simulink model "fivebar"  (R2018a)
settings: Solver=FixedStepAuto  StartTime=0.0  StopTime=1  FixedStep=10^-3  RelTol=1e-3  EnableMultiTasking=on
values from neighbouring files (symbols this model uses):
  ADAMS_cwd = '\\data-pfe\xshi2017\.Bureau\LAB3'    [Controls_Plant_6.m]    (also in Controls_Plant_7.m; Controls_Plant_8.m)
  ADAMS_exec = ''    [Controls_Plant_6.m]    (also in Controls_Plant_7.m; Controls_Plant_8.m)
  ADAMS_host = 'pc-b101-15.eleves.ecn'    [Controls_Plant_6.m]    (also in Controls_Plant_7.m; Controls_Plant_8.m)
  ADAMS_init = ''    [Controls_Plant_6.m]    (also in Controls_Plant_7.m; Controls_Plant_8.m)
  ADAMS_inputs = 'q11!q21'    [Controls_Plant_6.m]    (also in Controls_Plant_7.m; Controls_Plant_8.m)
  ADAMS_outputs = 'A13x!A13y!A13xd!A13yd!A13xdd!A13ydd!q12!q22!q13!q12d!q22d!q13d!q12dd!q22dd!q13dd!tau1!tau2'    [Controls_Plant_6.m]    (also in Controls_Plant_7.m; Controls_Plant_8.m)
  ADAMS_prefix = 'Controls_Plant_6'    [Controls_Plant_6.m]    (also in Controls_Plant_7.m = 'Controls_Plant_7'; Controls_Plant_8.m = 'Controls_Plant_8')
  ADAMS_static = 'no'    [Controls_Plant_6.m]    (also in Controls_Plant_7.m; Controls_Plant_8.m)
  ADAMS_sysdir = 'D:\Appli\Adams\'    [Controls_Plant_6.m]    (also in Controls_Plant_7.m; Controls_Plant_8.m)
settings Model: Creator=dsix  LastModifiedBy=xshi2017
settings DataIOCC: LimitDataPoints=on  SaveFormat=Array
settings OptimizationCC: LifeSpan=inf
settings DebuggingCC: SFUnexpectedBacktrackingDiag=warning  SFNoUnconditionalDefaultTransitionDiag=warning  SFExecutionAtInitializationDiag=none
settings HardwareCC: ProdBitPerPointer=32  ProdBitPerSizeT=32  ProdBitPerPtrDiffT=32  ProdLargestAtomicFloat=None  ProdIntDivRoundTo=Undefined  ProdEndianess=Unspecified  ProdWordSize=32  ProdHWDeviceType=32-bit Generic
settings ModelReferenceCC: PropagateSignalLabelsOutOfModel=off
settings CodeAppCC: StateflowObjectComments=on
settings GRTTargetCC: TargetLangStandard=C89/C90 (ANSI)  GeneratePreprocessorConditionals=Disable all
settings ConfigComp: CovMetricSettings=dw  CovHtmlReporting=on  CovSaveCumulativeToWorkspaceVar=on  CovSaveSingleToWorkspaceVar=on  CovExternalEMLEnable=off

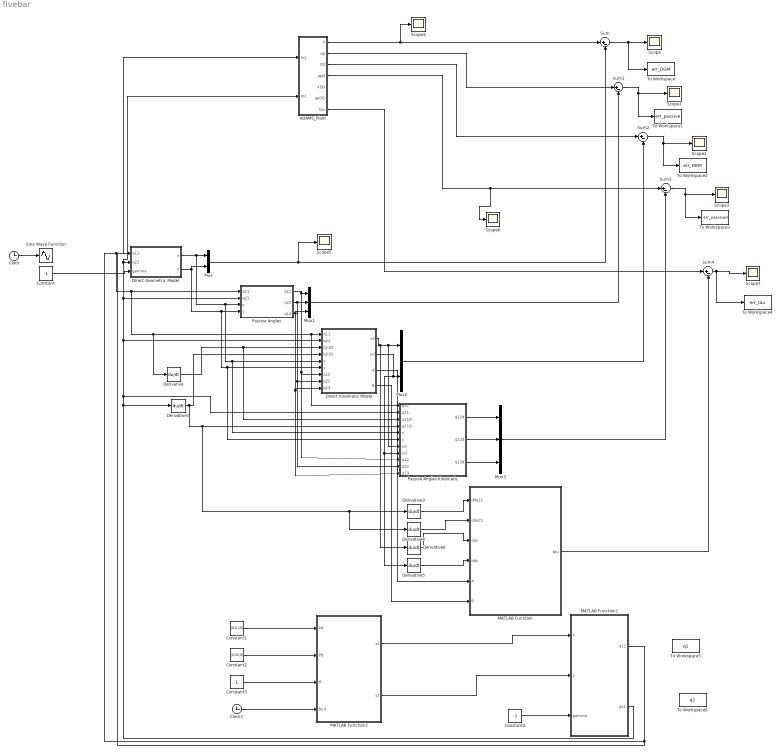
== system fivebar ==
  ADAMS_Plant : Subsystem
  Clock : Clock
  Clock1 : Clock
  Constant : Constant  Value=-1
  Constant1 : Constant  Value=[0;0.15]
  Constant2 : Constant  Value=[0.05;0]
  Constant3 : Constant
  Constant4 : Constant  Value=-1
  Derivative{,1,3..6} (6 alike) : Derivative
  Direct Geometric Model : MATLAB Function  TreatAsAtomicUnit=on
  Direct Kinematic Model : MATLAB Function  TreatAsAtomicUnit=on
  MATLAB Function : MATLAB Function  TreatAsAtomicUnit=on
  MATLAB Function1 : MATLAB Function  TreatAsAtomicUnit=on
  MATLAB Function2 : MATLAB Function  TreatAsAtomicUnit=on
  Mux : Mux  Inputs=2
  Mux1 : Mux  Inputs=3
  Mux2 : Mux  Inputs=2
  Mux3 : Mux  Inputs=3
  Passive Angles : MATLAB Function  TreatAsAtomicUnit=on
  Passive Angles Kinematic : MATLAB Function  TreatAsAtomicUnit=on
  Scope{,1..7} (8 alike) : Scope
  Sine Wave Function : Sin  TimeSource=Use external signal  SampleTime=0
  Sum{,1..4} (5 alike) : Sum  Inputs=|+-
  To Workspace : ToWorkspace  VariableName=err_DGM  SaveFormat=Timeseries  SampleTime=-1
  To Workspace1 : ToWorkspace  VariableName=err_passive  SaveFormat=Timeseries  SampleTime=-1
  To Workspace2 : ToWorkspace  VariableName=err_DKM  SaveFormat=Timeseries  SampleTime=-1
  To Workspace3 : ToWorkspace  VariableName=err_passived  SaveFormat=Timeseries  SampleTime=-1
  To Workspace4 : ToWorkspace  VariableName=err_tau  SaveFormat=Timeseries  SampleTime=-1
  To Workspace5 : ToWorkspace  VariableName=q1  SaveFormat=Timeseries  SampleTime=-1
  To Workspace6 : ToWorkspace  VariableName=q2  SaveFormat=Timeseries  SampleTime=-1
  wires:
  ADAMS_Plant/1(X) -> Scope4/1, Sum/1
  Sum/1 -> To Workspace/1, Scope/1
  Direct Geometric Model/1(x) -> Direct Kinematic Model/5(x), Passive Angles Kinematic/5(x), Passive Angles/3(x), Mux/1
  Direct Geometric Model/2(y) -> Mux/2, Passive Angles Kinematic/6(y), Direct Kinematic Model/6(y), Passive Angles/4(y)
  Mux/1 -> Scope5/1, Sum/2
  Passive Angles/1(q12) -> Passive Angles Kinematic/9(q12), Direct Kinematic Model/7(q12), Mux1/1
  Passive Angles/2(q22) -> Passive Angles Kinematic/10(q22), Direct Kinematic Model/8(q22), Mux1/2
  Passive Angles/3(q13) -> Passive Angles Kinematic/11(q13), Direct Kinematic Model/9(q13), Mux1/3
  ADAMS_Plant/2(qp) -> Sum1/1
  Mux1/1 -> Sum1/2
  Sum1/1 -> To Workspace1/1, Scope1/1
  Direct Kinematic Model/1(xd) -> Derivative6/1, Passive Angles Kinematic/7(xd), Mux2/1
  Direct Kinematic Model/2(yd) -> Passive Angles Kinematic/8(yd), Derivative5/1, Mux2/2
  Sum2/1 -> To Workspace2/1, Scope2/1
  Mux2/1 -> Sum2/2
  ADAMS_Plant/3(XD) -> Sum2/1
  Passive Angles Kinematic/1(q12d) -> Mux3/1
  Passive Angles Kinematic/2(q22d) -> Mux3/2
  Passive Angles Kinematic/3(q13d) -> Mux3/3
  Sum3/1 -> To Workspace3/1, Scope3/1
  Mux3/1 -> Sum3/2
  ADAMS_Plant/4(qpD) -> Scope6/1, Sum3/1
  MATLAB Function1/1(q11) -> Direct Geometric Model/1(q11), Derivative/1, Passive Angles Kinematic/1(q11), Direct Kinematic Model/1(q11), Passive Angles/1(q11), ADAMS_Plant/1(In1)
  Derivative/1 -> Passive Angles Kinematic/3(q11D), Direct Kinematic Model/3(q11D)
  Derivative1/1 -> Derivative4/1, Derivative3/1, Passive Angles Kinematic/4(q21D), Direct Kinematic Model/4(q21D)
  Derivative3/1 -> MATLAB Function/1(ddq11)
  Derivative5/1 -> MATLAB Function/4(ddy)
  Derivative6/1 -> MATLAB Function/3(ddx)
  Direct Kinematic Model/4(B) -> MATLAB Function/6(B)
  Direct Kinematic Model/3(A) -> MATLAB Function/5(A)
  ADAMS_Plant/7(tau) -> Sum4/1
  MATLAB Function/1(tau) -> Sum4/2
  Sum4/1 -> To Workspace4/1, Scope7/1
  Derivative4/1 -> MATLAB Function/2(ddq21)
  Constant1/1 -> MATLAB Function2/1(PA)
  Constant2/1 -> MATLAB Function2/2(PB)
  Constant3/1 -> MATLAB Function2/3(tf)
  Clock1/1 -> MATLAB Function2/4(tout)
  Constant4/1 -> MATLAB Function1/3(gamma)
  Clock/1 -> Sine Wave Function/1
  MATLAB Function2/2(yt) -> MATLAB Function1/2(y)
  MATLAB Function2/1(xt) -> MATLAB Function1/1(x)
  Constant/1 -> Direct Geometric Model/3(gamma)
  MATLAB Function1/2(q21) -> Derivative1/1, Passive Angles Kinematic/2(q21), Direct Kinematic Model/2(q21), Passive Angles/2(q21), ADAMS_Plant/2(In2), Direct Geometric Model/2(q21)

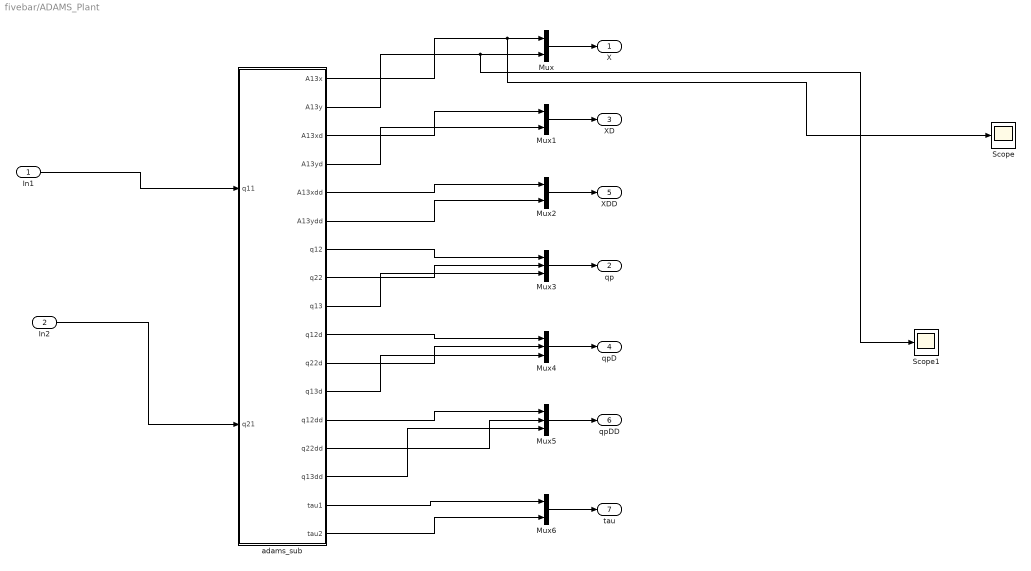
== system fivebar/ADAMS_Plant ==
  In1 : Inport
  In2 : Inport  Port=2
  Mux{,1..2,6} (4 alike) : Mux  Inputs=2
  Mux3 : Mux  Inputs=3
  Mux4 : Mux  Inputs=3
  Mux5 : Mux  Inputs=3
  Scope : Scope
  Scope1 : Scope
  adams_sub : Subsystem
  X : Outport
  qp : Outport  Port=2
  XD : Outport  Port=3
  qpD : Outport  Port=4
  XDD : Outport  Port=5
  qpDD : Outport  Port=6
  tau : Outport  Port=7
  wires:
  Mux1/1 -> XD/1
  Mux/1 -> X/1
  Mux2/1 -> XDD/1
  Mux5/1 -> qpDD/1
  Mux4/1 -> qpD/1
  Mux3/1 -> qp/1
  Mux6/1 -> tau/1
  In1/1 -> adams_sub/1(q11)
  In2/1 -> adams_sub/2(q21)
  adams_sub/1("A13x  ") -> Scope/1, Mux/1
  adams_sub/2("A13y  ") -> Scope1/1, Mux/2
  adams_sub/3("A13xd ") -> Mux1/1
  adams_sub/4("A13yd ") -> Mux1/2
  adams_sub/5(A13xdd) -> Mux2/1
  adams_sub/6(A13ydd) -> Mux2/2
  adams_sub/7("q12   ") -> Mux3/1
  adams_sub/8("q22   ") -> Mux3/2
  adams_sub/9("q13   ") -> Mux3/3
  adams_sub/10("q12d  ") -> Mux4/1
  adams_sub/11("q22d  ") -> Mux4/2
  adams_sub/12("q13d  ") -> Mux4/3
  adams_sub/13("q12dd ") -> Mux5/1
  adams_sub/14("q22dd ") -> Mux5/2
  adams_sub/15("q13dd ") -> Mux5/3
  adams_sub/16("tau1  ") -> Mux6/1
  adams_sub/17("tau2  ") -> Mux6/2

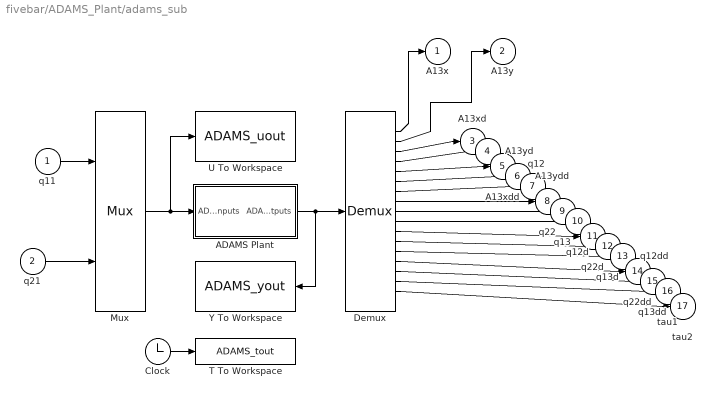
== system fivebar/ADAMS_Plant/adams_sub ==
  q11 : Inport
  q21 : Inport  Port=2
  ADAMS Plant : Subsystem  LoadFcn=|  InitFcn=clear mex  mask(Adams Plant){exevie=ADAMS_sysdir, nam_in=ADAMS_inputs, namout=ADAMS_outputs, nampre=ADAMS_prefix, outfil=ADAMS_prefix, exesol=ADAMS_exec, stat=ADAMS_static, inicmd=[ADAMS_init], exetyp=C++, comtyp=PIPE(DDE), workdir=ADAMS_cwd, ada_host=ADAMS_host, modani=interactive, modsim=discrete, dft=no, simulink_lead_cosim=yes, pin_interp_order=0, pout_extrap_order=0, pin_extrap_order=0, pout_interp_order=0, dt_out=0.005, o_rate=1, more=off}
      | %check based on dialog box setting for when setting by popup menu                                             
      | if exist('ADAMS_solver_type')                                                                                 
      |   if strcmp(ADAMS_solver_type,'C++')                                                                          
      |     set_param(gcb,'exetyp','C++');                                                                            
      |   else                                                                                                        
      |     set_param(gcb,'exetyp','Fortran');                                                                        
      |   end                                                                                                         
      | else                                                                                                          
      |   set_param(gcb,'exetyp','C++');                                                                              
      | end                                                                                                           
      | %set the mode if using acar_solver                                                                            
      | %REQUIRED HERE BECAUSE BELOW CAUSES MDLTERMINATE TO BE CALLED 2 TIMES IN MIDDLE OF SIMULATION WHEN SET IN MASK
      |                                                                                                               
      | %enable the direct feedthrough, sim mode, anim mode parameters by default                                     
      |                                                                                                               
      | if exist('set_some_params_states')                                                                            
      |                                                                                                               
      |   set_some_params_states({'dft','modsim','modani'},{'on','on','on'},'MaskEnables',gcb)                        
      |   %turn on direct feedthrough option                                                                          
      |   set_some_params_states({'dft'},{'on'},'MaskVisibilities',gcb)                                               
      |                                                                                                               
      |  end                                                                                                          
      |                                                                                                               
      |                                                                                                               
      | if exist('ADAMS_exec')                                                                                        
      |   if and(strcmp(get_param(gcb,'exesol'),'ADAMS_exec'),strcmp(ADAMS_exec,'acar_solver'))                       
      |     %set the sim mode to discrete -- only supported mode                                                      
      |     set_param(gcb,'modsim','discrete')                                                                        
      |      %turn off direct feedthrough option                                                                      
      |      set_some_params_states({'dft'},{'off'},'MaskVisibilities',gcb)                                           
      |     %set the animation mode to batch -- only supported mode                                                   
      |     set_param(gcb,'modani','batch')                                                                           
      |     %disable the direct feedthrough, sim mode, anim mode parameters                                           
      |     set_some_params_states({'modsim','modani'},{'off','off'},'MaskEnables',gcb)                               
      |   end                                                                                                         
      | end
      mask prompts: exevie "Adams install directory"; nam_in "Adams/View input names"; namout "Adams/View output names"; nampre "Adams model file prefix"; outfil "Output files prefix (opt.: if blank - no output)"; exesol "User executable (opt.: if blank - use standard)"; stat "Initial static simulation flag"; inicmd "Initialization commands"; exetyp "Adams/Solver type"; comtyp "Interprocess option"; workdir "Adams working directory"; ada_host "Adams host"; modani "Animation mode"; modsim "Simulation mode"; dft "Direct feedthrough"; simulink_lead_cosim "Discrete Computational Order - Simulink Leads Adams"; pin_interp_order "Plant input interpolation order"; pout_extrap_order "Plant output extrapolation order"; pin_extrap_order "Plant input extrapolation order"; pout_interp_order "Plant output interpolation order"; dt_out "Communication interval"; o_rate "Number of communications per output step"; more "More parameters"
      mask help: Simulate any Adams plant model either in Adams/Solver form (.adm file) or in Adams/View form (.cmd file)
      settings: OpenFcn=|
      | open_system(gcb,'mask')
      | if not(exist('set_some_params_states'))
      | 
      | warning('The script "set_some_params_states.m" cannot be found in the MATLAB PATH.  Cannot update the ADAMS Plant S-Function parameters.')
      | 
      | warning('Recommended action(optional):  run the Adams/Controls .m file first to help choose the correct settings in the Adams S-Function block.')
      | 
      | end
      mask Help:
      | <html>
      | This S-Function represents the non-linear Adams Plant with the inputs sent to the Adams model <br>
      |  and the outputs generated by the Adams model.  See the Adams/Controls documentation for more <br>
      | information.  This plant uses the following variables:<br>
      | <br>
      | <b>ADAMS_sysdir  :</b> Adams installation directory<br>
      | <b>ADAMS_inputs  :</b> Input variables View names vector<br>
      | <b>ADAMS_outputs :</b> Outputs variables View names vector<br>
      | <b>ADAMS_prefix  : </b>ADAMS model files prefix (.adm, .cmd); also doubles as output files prefix<br>
      | <b>ADAMS_exec :</b> Adams/Solver user library or keyword (e.g., acar_solver)<br>
      | <b>ADAMS_static :</b> yes|no - initial static before Co-simulation(discrete)/Function Evaluation(continuous)<br>
      | <b>ADAMS_init :</b>Initialization commands (i.e., Adams/View or Solver commands, depending on setting for Animation mode)<br>
      | <b>ADAMS_cwd : </b> Current working directory (for TCP/IP)<br>
      | <b>ADAMS_host : </b>Name of Adams server host (for TCP/IP)<br>
      | <b>ADAMS_mode :</b> Linear or non-linear (i.e., co-sim, function eval)<br>
      | <b>ADAMS_solver_type :</b>Fortran or C++ (used to set popup menu when first loaded) <br>
      | 
      | 
      | <br>
      | The following settings can be chosen:<br>
      | <br>
      | <b>Adams/Solver type:</b>  Fortran or C++ (will also set ADAMS_solver_type)<br>
      | <b>Interprocess option:</b> Pipe(DDE) or TCP/IP; TCP/IP can allow different machines run Adams and MATLAB<br>
      | <b>Animation mode:</b> batch (Solver, uses .adm) or interactive (View, uses .cmd)<br>
      | <b>Simulation mode:</b> discrete (Co-simulation) or continuous (Function Evaluation)<br>
      | <b>Discrete Computational Order - Simulink Lead Adams:</b> for discrete mode, chooses if Simulink leads the integration (yes) or lags (no);<br> if set to "no", can remove algebraic loop<br>
      | <b>Plant input interpolation order:</b> 0 = zero-order hold; 1 = linear (discrete mode only, where Simulink leads)<br>
      | <b>Plant output extrapolation order:</b> 0 = zero-order hold;1 = linear(discrete mode only, where Simulink leads)<br>
      | <b>Plant input extrapolation order:</b> 0 = zero-order hold; 1 = linear (discrete mode only, where Adams leads)<br>
      | <b>Plant output interpolation order:</b> 0 = zero-order hold;1 = linear(discrete mode only, where Adams leads)<br>
      | <b>Direct feedthrough:</b> yes|no - yes = Input directly effect output(continuous mode-only)<br>
      | <b>Communication interval:</b> Time step at which Co-simulation exchange information (e.g.,0.005); also controls <br>output for continuous mode (Function Evaluation)<br>
      | <b>Number of communications per output step: </b>Sets Adams output rate (.res, .req, .gra) integer value (default: 1)<br>
      | </html>
      mask Callback exesol:
      | if exist('set_some_params_states')
      | %enable the direct feedthrough, sim mode, anim mode parameters
      | set_some_params_states({'dft','modsim','modani'},{'on','on','on'},'MaskEnables',gcb)
      | %turn on direct feedthrough option
      | set_some_params_states({'dft'},{'on'},'MaskVisibilities',gcb)
      | end
      | 
      | if exist('ADAMS_exec')
      |   if and(strcmp(get_param(gcb,'exesol'),'ADAMS_exec'),strcmp(ADAMS_exec,'acar_solver'))
      |     %set the sim mode to discrete -- only supported mode
      |     %REMOVED:  BELOW CAUSES MDLTERMINATE TO BE CALLED 2 TIMES IN MIDDLE OF SIMULATION
      |     %Now in LoadFcn callback
      |     %set_param(gcb,'modsim','discrete')
      |      %turn off direct feedthrough option
      |     set_some_params_states({'dft'},{'off'},'MaskVisibilities',gcb)
      |     %set the animation mode to batch -- only supported mode
      |     %REMOVED:  BELOW CAUSES MDLTERMINATE TO BE CALLED 2 TIMES IN MIDDLE OF SIMULATION
      |     %Now in LoadFcn callback
      |     %set_param(gcb,'modani','batch')
      |     %disable the direct feedthrough, sim mode, anim mode parameters
      |     set_some_params_states({'modsim','modani'},{'off','off'},'MaskEnables',gcb)
      |   end
      | end
      mask TypeOptions exetyp: Fortran | C++
      mask Callback exetyp:
      | if strcmp(get_param(gcb,'exetyp'),'C++')
      |     ADAMS_solver_type='C++';
      | else
      |     ADAMS_solver_type='Fortran';
      | end
      mask TypeOptions comtyp: PIPE(DDE) | TCP/IP
      mask Callback comtyp:
      | if exist('set_some_params_states')
      | if strcmp(get_param(gcb,'comtyp'),'PIPE(DDE)')
      |     %turn off cwd, host options
      |     set_some_params_states({'ada_host','workdir'},{'off','off'},'MaskVisibilities',gcb)
      | else%if strcmp(get_param(gcb,'modsim'),'TCP/IP')
      |     %turn on cwd, host options
      |     set_some_params_states({'ada_host','workdir'},{'on','on'},'MaskVisibilities',gcb)
      | end
      | end
      mask TypeOptions modani: batch | interactive
      mask TypeOptions modsim: discrete | continuous
      mask Callback modsim:
      | if exist('set_some_params_states')
      | if strcmp(get_param(gcb,'modsim'),'discrete')
      |      %turn off direct feedthrough option
      |     set_some_params_states({'dft'},{'off'},'MaskVisibilities',gcb)
      |     %turn on discrete co-sim type if want to see more
      |     if strcmp(get_param(gcb,'more'),'on')
      |         set_some_params_states({'simulink_lead_cosim'},{'on'},'MaskVisibilities',gcb)
      |     end
      |     if strcmp(get_param(gcb,'simulink_lead_cosim'),'yes')
      |         %turn on interpolation/extrapolation options
      |         set_some_params_states({'pin_interp_order','pout_extrap_order',},{'on','on'},'MaskVisibilities',gcb)
      |     else
      |         set_some_params_states({'pin_extrap_order','pout_interp_order'},{'on','on'},'MaskVisibilities',gcb)
      |     end
      | else%if strcmp(get_param(gcb,'modsim'),'continuous')
      |      %turn off direct feedthrough option
      |     set_some_params_states({'dft'},{'on'},'MaskVisibilities',gcb)
      |     %turn off interpolation/extrapolation options
      |     set_some_params_states({'pin_interp_order','pout_extrap_order','pin_extrap_order','pout_interp_order','simulink_lead_cosim'},{'off','off','off','off','off'},'MaskVisibilities',gcb)
      | end
      | end
      mask TypeOptions dft: no | yes
      mask TypeOptions simulink_lead_cosim: yes | no
      mask Callback simulink_lead_cosim:
      | if exist('set_some_params_states')
      | if (strcmp(get_param(gcb,'simulink_lead_cosim'),'yes') && strcmp(get_param(gcb,'modsim'),'discrete'))
      |      %turn off unused interpolate/extrapolate options
      |     set_some_params_states({'pin_extrap_order','pout_interp_order'},{'off','off'},'MaskVisibilities',gcb)
      |     %turn on used interpolate/extrapolate options
      |     set_some_params_states({'pin_interp_order','pout_extrap_order'},{'on','on'},'MaskVisibilities',gcb)
      | elseif (strcmp(get_param(gcb,'simulink_lead_cosim'),'no') && strcmp(get_param(gcb,'modsim'),'discrete'))
      |     %turn on used interpolate/extrapolate options
      |     set_some_params_states({'pin_extrap_order','pout_interp_order'},{'on','on'},'MaskVisibilities',gcb)
      |      %turn off unused interpolate/extrapolate options
      |     set_some_params_states({'pin_interp_order','pout_extrap_order'},{'off','off'},'MaskVisibilities',gcb)
      | end
      | end
      mask TypeOptions pin_interp_order: 0 | 1
      mask TypeOptions pout_extrap_order: 0 | 1
      mask TypeOptions pin_extrap_order: 0 | 1
      mask TypeOptions pout_interp_order: 0 | 1
      mask Callback more:
      | if exist('set_some_params_states')
      | if (strcmp(get_param(gcb,'more'),'on'))
      |      %turn on infrequently used options
      |     set_some_params_states({'exevie','nam_in','namout','exesol','stat','inicmd'},{'on','on','on','on','on','on'},'MaskVisibilities',gcb)
      |     if strcmp(get_param(gcb,'modsim'),'discrete')
      |         set_some_params_states({'simulink_lead_cosim'},{'on'},'MaskVisibilities',gcb)
      |     end
      | elseif (strcmp(get_param(gcb,'more'),'off'))
      |     %turn off infrequently used options
      |     set_some_params_states({'exevie','nam_in','namout','exesol','stat','inicmd'},{'off','off','off','off','off','off'},'MaskVisibilities',gcb)
      |     if strcmp(get_param(gcb,'modsim'),'discrete')
      |         set_some_params_states({'simulink_lead_cosim'},{'off'},'MaskVisibilities',gcb)
      |     end
      | end
      | end
      mask Display: disp( 'MSC Software' )
  Clock : Clock
  Demux : Demux  Outputs=17
  Mux : Mux  Inputs=2
  T To Workspace : ToWorkspace  VariableName=ADAMS_tout
      settings: MaxDataPoints=100000
  U To Workspace : ToWorkspace  VariableName=ADAMS_uout
      settings: MaxDataPoints=100000
  Y To Workspace : ToWorkspace  VariableName=ADAMS_yout
      settings: MaxDataPoints=100000
  "A13x  " : Outport
  "A13y  " : Outport  Port=2
  "A13xd " : Outport  Port=3
  "A13yd " : Outport  Port=4
  A13xdd : Outport  Port=5
  A13ydd : Outport  Port=6
  "q12   " : Outport  Port=7
  "q22   " : Outport  Port=8
  "q13   " : Outport  Port=9
  "q12d  " : Outport  Port=10
  "q22d  " : Outport  Port=11
  "q13d  " : Outport  Port=12
  "q12dd " : Outport  Port=13
  "q22dd " : Outport  Port=14
  "q13dd " : Outport  Port=15
  "tau1  " : Outport  Port=16
  "tau2  " : Outport  Port=17
  wires:
  Clock/1 -> T To Workspace/1
  Mux/1 -> ADAMS Plant/1(ADAMS inputs), U To Workspace/1
  ADAMS Plant/1(ADAMS outputs) -> Demux/1, Y To Workspace/1
  Demux/1 -> "A13x  "/1
  Demux/2 -> "A13y  "/1
  Demux/3 -> "A13xd "/1
  Demux/4 -> "A13yd "/1
  Demux/5 -> A13xdd/1
  Demux/6 -> A13ydd/1
  Demux/7 -> "q12   "/1
  Demux/8 -> "q22   "/1
  Demux/9 -> "q13   "/1
  Demux/10 -> "q12d  "/1
  Demux/11 -> "q22d  "/1
  Demux/12 -> "q13d  "/1
  Demux/13 -> "q12dd "/1
  Demux/14 -> "q22dd "/1
  Demux/15 -> "q13dd "/1
  Demux/16 -> "tau1  "/1
  Demux/17 -> "tau2  "/1
  q11/1 -> Mux/1
  q21/1 -> Mux/2

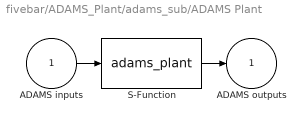
== system fivebar/ADAMS_Plant/adams_sub/ADAMS Plant ==
  ADAMS inputs : Inport
  S-Function : S-Function  StopFcn=clear mex  FunctionName=adams_plant  Parameters=exevie,exesol,stat,outfil,nampre,o_rate,nam_in,namout,dft,modsim,modani,dt_out,inicmd,exetyp,comtyp,ada_host, workdir,pin_interp_order,pout_extrap_order,pin_extrap_order,pout_interp_order,simulink_lead_cosim  SFunctionDeploymentMode=off  EnableBusSupport=off
  ADAMS outputs : Outport  InitialOutput=0
  wires:
  ADAMS inputs/1 -> S-Function/1
  S-Function/1 -> ADAMS outputs/1

== matlab function fivebar/Passive Angles ==
  data: q11 input; q12 output; q21 input; x input; q22 output; q13 output; y input
function [q12,q22,q13] = passive_angles(q11,q21,x,y)
d = 0.118;
l = 0.09;
% A11 = [-d/2;0];
% A21 = [d/2;0];
% A12 = [-d/2+cos(q11)*l;sin(q11)*l];
% A22 = [d/2+cos(q21)*l;sin(q21)*l];
% A13 = [x;y];

% q12 = acos(dot((A12-A11),(A13-A12))/(norm(A12-A11)*norm(A13-A12)));
% q22 = acos(dot((A22-A21),(A13-A22))/(norm(A22-A21)*norm(A13-A22)));
% q13 = acos(dot((A13-A12),(A13-A22))/(norm(A13-A22)*norm(A13-A12)));

q12 = -q11 + atan2((y - l*sin(q11)),(x + d/2 - l*cos(q11)));

q22 = -q21 + atan2((y - l*sin(q21)),(x - d/2 - l*cos(q21)));

q13 = - q11 + q22 - q12 + q21;

end

== matlab function fivebar/Direct Geometric Model ==
  data: q11 input; x output; q21 input; gamma input; y output
function [x, y] = DGM(q11, q21, gamma)
d = 0.118;
l = 0.09;
A11 = [-d/2;0];
A21 = [d/2;0];
A12 = [-d/2+cos(q11)*l;sin(q11)*l];
A22 = [d/2+cos(q21)*l;sin(q21)*l];
A22H = (A12 - A22)/2;
a = norm(A22H);
h = abs(sqrt(l^2-a^2));
HA13 = gamma*(h/a)*[0,-1;1,0]*A22H;
E = A22 + A22H + HA13 ;
x = E(1);
y = E(2);
end

== matlab function fivebar/Direct Kinematic Model ==
  data: q11 input; q21 input; q11D input; q21D input; x input; y input; q12 input; q22 input; q13 input; xd output; yd output; A output; B output
function [xd,yd,A,B] = DKM(q11,q21,q11D,q21D,x,y,q12,q22,q13)

d = 0.118;
l = 0.09;
% A11 = [-d/2;0];
% A21 = [d/2;0];
% A12 = [-d/2+cos(q11)*l;sin(q11)*l];
% A22 = [d/2+cos(q21)*l;sin(q21)*l];
% A13 = [x;y];

v1 = [cos(q11+q12);sin(q11+q12)];
u1 = [cos(q11);sin(q11)];
v2 = [cos(q21+q22);sin(q21+q22)];
u2 = [cos(q21);sin(q21)];

E = [0 -1;1 0];

pd = inv([v1';v2'])*[l*sin(q12),0;0,l*sin(q22)]*[q11D;q21D];
xd = pd(1);
yd = pd(2);

A = [v1';v2'];

B = [l*sin(q12),0;0,l*sin(q22)];
end

== matlab function fivebar/Passive Angles Kinematic ==
  data: q11 input; q21 input; q11D input; q21D input; x input; y input; xd input; yd input; q12 input; q22 input; q13 input; q12d output; q22d output; q13d output
function [q12d,q22d,q13d] = passive_angleskm(q11,q21,q11D,q21D,x,y,xd,yd,q12,q22,q13)
d = 0.118;
l = 0.09;
% q12d = diff(q12);
E = [0 -1;1 0];

v1 = [cos(q11+q12);sin(q11+q12)];
u1 = [cos(q11);sin(q11)];
v2 = [cos(q21+q22);sin(q21+q22)];
u2 = [cos(q21);sin(q21)];

qd = inv([l,0;0,l]) * ([(E*v1)';(E*v2)']*[xd;yd] - [l*cos(q12)+l,0;0,l*cos(q22)+l]*[q11D;q21D]);
q12d = qd(1);
q22d = qd(2);
q13d =  - q11D + q22d - q12d + q21D;
end

== matlab function fivebar/MATLAB Function ==
  data: tau output; ddq11 input; ddq21 input; ddx input; ddy input; A input; B input
function tau = IDM(ddq11,ddq21,ddx,ddy,A,B)

zz11R = 0.013704725227;
zz21R = 0.014534710433;
m = 0.5071616221;

tau_a = [zz11R * ddq11 ;
     zz21R * ddq21];

tau_d = [0;
     0];

w_r = [m * ddx;
    m * ddy];

J = -A^-1 * B;

J_d = [0 0;
    0 0];

tau = tau_a + J * w_r + J_d' * tau_d;



end

== matlab function fivebar/MATLAB Function1 ==
  data: x input; q11 output; y input; q21 output; gamma input
function [q11,q21] = IGM(x,y,gamma)

d = 0.118;
l = 0.09;
A11H = [x/2+d/4;y/2];
A21H = [x/2-d/4;y/2];
h1 = norm(A11H);
h2 = norm(A21H);

a1 = abs(sqrt(l^2-h1^2));
a2 = abs(sqrt(l^2-h2^2));

q11 = -atan((1/2*x + d/4 + gamma * h1 /(2 * a1) * y)/(y/2 - (d / 4 + x / 2)*gamma * h1 / a1));

q21 = -atan((1/2*x - d/4 + gamma * h2 /(2 * a2) * y)/(y/2 - (-d / 4 + x / 2)*gamma * h2 / a2));

end

== matlab function fivebar/MATLAB Function2 ==
  data: PA input; xt output; PB input; tf input; tout input; yt output
function [xt,yt] = Dtrajectory(PA,PB,tf,tout)

s = 10*(tout/tf)^3 - 15*(tout/tf)^4 + 6*(tout/tf)^5;

xt = PA(1) + s*(PB(1) - PA(1));

yt = PA(2) + s*(PB(2) - PA(2));


end
